simulink model "publisher_task"  (Simulink 3.0)
libraries: stringlib x3, mathlib x2, logiclib x1, genlib x1, mqttlib x1

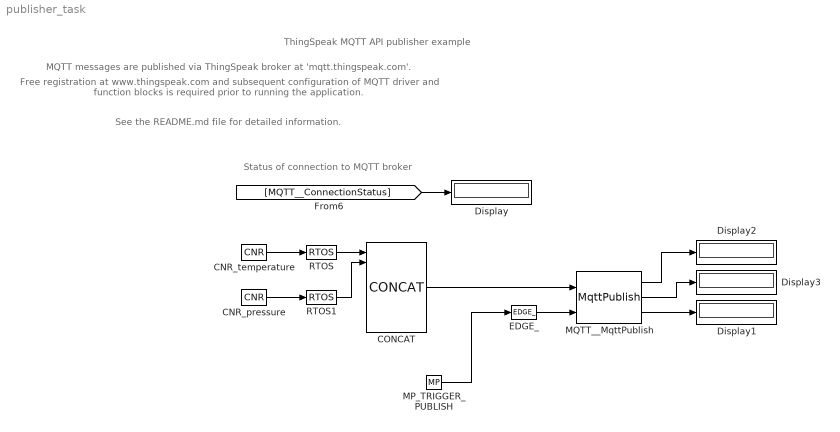
== system publisher_task ==
  note: Status of connection to MQTT broker
  note: ThingSpeak MQTT API publisher example
  note: MQTT messages are published via ThingSpeak broker at 'mqtt.thingspeak.com'.
  note: Free registration at www.thingspeak.com and subsequent configuration of MQTT
      | driver and function blocks is required prior to running the application.
  note: See the README.md file for detailed information.
  CNR_pressure : mathlib/CNR  ycn=104
  CNR_temperature : mathlib/CNR  ycn=9.81
  CONCAT : stringlib/CONCAT  ptrn=field1=%1&field2=%2  nmax=0
  Display{,1..3} (4 alike) : Display
      settings: Format=Best fit
  EDGE_ : logiclib/EDGE_  iedge=1: Rising edge
  MP_TRIGGER_PUBLISH : genlib/MP  BSTATE=off  pwidth=1  RPTF=off
  MQTT__MqttPublish : mqttlib/MqttPublish  topic=channels/<channelID>/publish/<WriteAPIKey>  QoS=1: QoS0 (At most once)  RETAIN=off  defBuffSize=80
  RTOS : stringlib/RTOS  prec=3  mode=2: normal
  RTOS1 : stringlib/RTOS  prec=0  mode=2: normal
  wires:
  CNR_pressure/1 -> RTOS1/1
  CNR_temperature/1 -> RTOS/1
  CONCAT/1 -> MQTT__MqttPublish/1
  EDGE_/1 -> MQTT__MqttPublish/2
  [MQTT__ConnectionStatus] -> Display/1
  MP_TRIGGER_PUBLISH/1 -> EDGE_/1
  MQTT__MqttPublish/1 -> Display2/1
  MQTT__MqttPublish/2 -> Display3/1
  MQTT__MqttPublish/3 -> Display1/1
  RTOS/1 -> CONCAT/1
  RTOS1/1 -> CONCAT/2
